simulink model "TerrainAwarePlanner"  (R2024a)
settings: Solver=FixedStepAuto  StartTime=0.0  StopTime=.1  RelTol=1e-3
undefined symbols (not defined in the file or in its folder): fixedTerrainAwareParams, maxRefPathLen
settings Model: Creator=cstabile  LastModifiedBy=cstabile
settings SFSimCC: MATLABDynamicMemAllocThreshold=10000000  SimTargetLang=C++
settings RTWCC: GPUComputeCapability=3.5

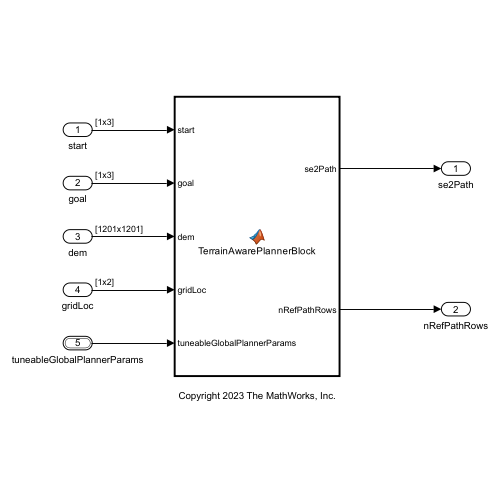
[thumbnail: Simulink's stored preview of the top-level diagram]
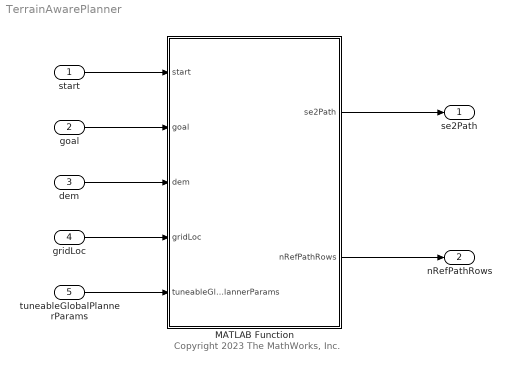
== system TerrainAwarePlanner ==
  note: Copyright 2023 The MathWorks, Inc.
  start : Inport  PortDimensions=[1 3]  Interpolate=off
  goal : Inport  Port=2  PortDimensions=[1 3]
  dem : Inport  Port=3  PortDimensions=[1201 1201]
  gridLoc : Inport  Port=4  PortDimensions=[1 2]
  tuneableGlobalPlannerParams : Inport  Port=5  OutDataTypeStr=Bus: fsp_tunable_bus
  MATLAB Function : MATLAB Function  TreatAsAtomicUnit=on  mask{length=fixedTerrainAwareParams.Length, width=fixedTerrainAwareParams.Width, numMotionPrimitives=fixedTerrainAwareParams.NumMotionPrimitives, analyticExpansionInterval=fixedTerrainAwareParams.AnalyticExpansionInterval, interpolationDistance=fixedTerrainAwareParams.InterpolationDistance, numCircles=fixedTerrainAwareParams.NumCircles, resolution=fixedTerrainAwareParams.Resolution, visualizePlanner=1, nRowOutput=maxRefPathLen}
      mask prompts: visualizePlanner "Visualize Planner"; nRowOutput "Maximum rows in output"
  se2Path : Outport
  nRefPathRows : Outport  Port=2
  wires:
  start/1 -> MATLAB Function/1(start)
  goal/1 -> MATLAB Function/2(goal)
  dem/1 -> MATLAB Function/3(dem)
  gridLoc/1 -> MATLAB Function/4(gridLoc)
  tuneableGlobalPlannerParams/1 -> MATLAB Function/5(tuneableGlobalPlannerParams)
  MATLAB Function/1(se2Path) -> se2Path/1
  MATLAB Function/2(nRefPathRows) -> nRefPathRows/1

== matlab function TerrainAwarePlanner/MATLAB Function ==
  data: start input size=[1 3]; se2Path output size=[nRowOutput 3]; goal input size=[1 3]; dem input single; gridLoc input; tuneableGlobalPlannerParams input; length parameter size=[1 1]; width parameter size=[1 1]; resolution parameter size=[1 1]; numMotionPrimitives parameter; analyticExpansionInterval parameter; numCircles parameter; nRefPathRows output; nRowOutput parameter
function [se2Path,nRefPathRows] = TerrainAwarePlannerBlock(start,goal,dem,gridLoc,tuneableGlobalPlannerParams,length, width, resolution, numMotionPrimitives, analyticExpansionInterval, numCircles, nRowOutput)
    fixedParams = struct( ...
        'Length',coder.const(length), ...
        'Width',coder.const(width), ...
        'NumMotionPrimitives',numMotionPrimitives, ...
        'AnalyticExpansionInterval',analyticExpansionInterval, ...
        'NumCircles',numCircles, ...
        'Resolution',resolution);
    
    % Convert world coordinates to local coordinates since costmap cannot
    % update its location during codegen
    localStart = start - [gridLoc 0];
    localGoal = goal - [gridLoc 0];
    se2Path_ = TerrainAwarePlannerFcn(localStart,localGoal,dem,gridLoc,tuneableGlobalPlannerParams,fixedParams);
    se2Path = zeros(nRowOutput,3);
    nRefPathRows = size(se2Path_,1);
    se2Path(1:nRefPathRows,:) = se2Path_+[gridLoc 0];
end
